simulink subsystem "VehicleBody6DOFSSC"  (R2023b)
settings: Solver=VariableStepAuto  StartTime=0.0  StopTime=10.0  RelTol=1e-3
undefined symbols (not defined in the file): EnvAirDen, PlntVehAeroDragCff, PlntVehAeroFrntArea, PlntVehAeroLiftCff, PlntVehCGHgtAxl, PlntVehDstCGFrntAxl, PlntVehDstCGRearAxl, PlntVehInitLatPos, PlntVehInitVertPos, PlntVehMass, PlntVehMultiBody, PlntVehPitchMomentInertia, PlntVehRollMomentInertia, PlntVehYawMomentInertia, X, Y, Z
libraries: nesl_utility x44, sm_lib x42, sharedtransform x12, fl_lib x4, vehdynlibeomcommon x3, matrix_library x1
(part 2 of 3)

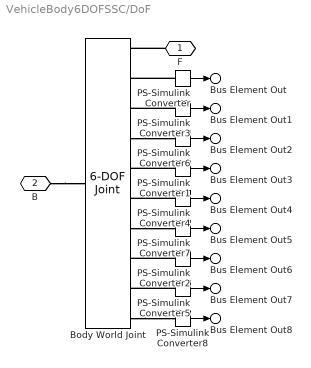
== system VehicleBody6DOFSSC/DoF ==
  Body World Joint : sm_lib/Joints/6-DOF Joint  JointMode=Normal  SenseConstraintForce=off  SenseConstraintForceX=off  SenseConstraintForceY=off  SenseConstraintForceZ=off  SenseConstraintTorque=off  SenseConstraintTorqueX=off  SenseConstraintTorqueY=off  SenseConstraintTorqueZ=off  SenseTotalForce=off  SenseTotalForceX=off  SenseTotalForceY=off  SenseTotalForceZ=off  SenseTotalTorque=off  SenseTotalTorqueX=off  SenseTotalTorqueY=off  SenseTotalTorqueZ=off  CompositeWrenchDir=FollowerOnBase  CompositeWrenchFrame=BaseFrame  PxEquilibriumPosition=0  PxEquilibriumPositionUnits=m  PxSpringStiffness=0  PxSpringStiffnessUnits=N/m  PxDampingCoefficient=0  PxDampingCoefficientUnits=N/(m/s)  PxTorqueActuationMode=NoTorque  PxMotionActuationMode=ComputedMotion  PxSensePosition=on  PxSenseVelocity=on  PxSenseAcceleration=on  PxSenseTorqueForce=off  PxSenseLowerLimitTorqueForce=off  PxSenseUpperLimitTorqueForce=off  PxLowerLimitSpecify=off  PxLowerLimitBound=-1  PxLowerLimitBoundUnits=m  PxLowerLimitStiffness=1e6  PxLowerLimitStiffnessUnits=N/m  PxLowerLimitDamping=1e3  PxLowerLimitDampingUnits=N/(m/s)  PxLowerLimitTransitionRegionWidth=1e-4  PxLowerLimitTransitionRegionWidthUnits=m  PxUpperLimitSpecify=off  PxUpperLimitBound=1  PxUpperLimitBoundUnits=m  PxUpperLimitStiffness=1e6  PxUpperLimitStiffnessUnits=N/m  PxUpperLimitDamping=1e3  PxUpperLimitDampingUnits=N/(m/s)  PxUpperLimitTransitionRegionWidth=1e-4  PxUpperLimitTransitionRegionWidthUnits=m  PxPositionTargetSpecify=on  PxPositionTargetPriority=Low  PxPositionTargetValue=PlntVehInitLongPos  PxPositionTargetValueUnits=m  PxVelocityTargetSpecify=on  PxVelocityTargetPriority=Low  PxVelocityTargetValue=0  PxVelocityTargetValueUnits=m/s  PyEquilibriumPosition=0  PyEquilibriumPositionUnits=m  PySpringStiffness=0  PySpringStiffnessUnits=N/m  PyDampingCoefficient=0  PyDampingCoefficientUnits=N/(m/s)  PyTorqueActuationMode=NoTorque  PyMotionActuationMode=ComputedMotion  PySensePosition=on  PySenseVelocity=on  PySenseAcceleration=on  PySenseTorqueForce=off  PySenseLowerLimitTorqueForce=off  PySenseUpperLimitTorqueForce=off  PyLowerLimitSpecify=off  PyLowerLimitBound=-1  PyLowerLimitBoundUnits=m  PyLowerLimitStiffness=1e6  PyLowerLimitStiffnessUnits=N/m  PyLowerLimitDamping=1e3  PyLowerLimitDampingUnits=N/(m/s)  PyLowerLimitTransitionRegionWidth=1e-4  PyLowerLimitTransitionRegionWidthUnits=m  PyUpperLimitSpecify=off  PyUpperLimitBound=1  PyUpperLimitBoundUnits=m  PyUpperLimitStiffness=1e6  PyUpperLimitStiffnessUnits=N/m  PyUpperLimitDamping=1e3  PyUpperLimitDampingUnits=N/(m/s)  PyUpperLimitTransitionRegionWidth=1e-4  PyUpperLimitTransitionRegionWidthUnits=m  PyPositionTargetSpecify=on  PyPositionTargetPriority=Low  PyPositionTargetValue=-PlntVehInitLatPos  PyPositionTargetValueUnits=m  PyVelocityTargetSpecify=on  PyVelocityTargetPriority=Low  PyVelocityTargetValue=0  PyVelocityTargetValueUnits=m/s  PzEquilibriumPosition=0  PzEquilibriumPositionUnits=m  PzSpringStiffness=0  PzSpringStiffnessUnits=N/m  PzDampingCoefficient=0  PzDampingCoefficientUnits=N/(m/s)  PzTorqueActuationMode=NoTorque  PzMotionActuationMode=ComputedMotion  PzSensePosition=on  PzSenseVelocity=on  PzSenseAcceleration=on  PzSenseTorqueForce=off  PzSenseLowerLimitTorqueForce=off  PzSenseUpperLimitTorqueForce=off  PzLowerLimitSpecify=off  PzLowerLimitBound=-1  PzLowerLimitBoundUnits=m  PzLowerLimitStiffness=1e6  PzLowerLimitStiffnessUnits=N/m  PzLowerLimitDamping=1e3  PzLowerLimitDampingUnits=N/(m/s)  PzLowerLimitTransitionRegionWidth=1e-4  PzLowerLimitTransitionRegionWidthUnits=m  PzUpperLimitSpecify=off  PzUpperLimitBound=1  PzUpperLimitBoundUnits=m  PzUpperLimitStiffness=1e6  PzUpperLimitStiffnessUnits=N/m  PzUpperLimitDamping=1e3  PzUpperLimitDampingUnits=N/(m/s)  PzUpperLimitTransitionRegionWidth=1e-4  PzUpperLimitTransitionRegionWidthUnits=m  PzPositionTargetSpecify=on  PzPositionTargetPriority=Low  PzPositionTargetValue=-PlntVehInitVertPos*0  PzPositionTargetValueUnits=m  PzVelocityTargetSpecify=on  PzVelocityTargetPriority=Low  PzVelocityTargetValue=0  PzVelocityTargetValueUnits=m/s  SphEqPosRotationMethod=None  SphEqPosRotationAngleUnits=deg  SphEqPosRotationStandardAxis=+Z  SphEqPosRotationAngle=0.0  SphEqPosRotationArbitraryAxis=[0 0 1]  SphEqPosFollAlignAxisA=+X  SphEqPosBaseAlignAxisA=+Y  SphEqPosFollAlignAxisB=+Y  SphEqPosBaseAlignAxisB=+Z  SphEqPosRotationSequenceAxes=FollowerAxes  SphEqPosRotationSequence=XYX  SphEqPosRotationSequenceAngles=[0 0 0]  SphEqPosRotationSequenceAnglesUnits=deg  SphEqPosRotationMatrix=[1 0 0; 0 1 0; 0 0 1]  SphEqPosQuaternion=[1 0 0 0]  SphSpringStiffness=0  SphSpringStiffnessUnits=N*m/deg  SphDampingCoefficient=0  SphDampingCoefficientUnits=N*m/(deg/s)  SphActuateTorqueX=off  SphActuateTorqueY=off  SphActuateTorqueZ=off  SphActuateTorque=off  SphTorqueActuationMode=NoTorque  SphMotionActuationMode=ComputedMotion  SphActuationFrame=BaseFrame  SphSensePosition=off  SphSenseVelocityX=off  SphSenseVelocityY=off  SphSenseVelocityZ=off  SphSenseVelocity=off  SphSenseAccelerationX=off  SphSenseAccelerationY=off  SphSenseAccelerationZ=off  SphSenseAcceleration=off  SphSenseTorqueX=off  SphSenseTorqueY=off  SphSenseTorqueZ=off  SphSenseTorqueForce=off  SphSenseLowerLimitTorqueMag=off  SphSenseUpperLimitTorqueMag=off  SphSensingFrame=BaseFrame  SphLowerLimitSpecify=off  SphLowerLimitBound=15  SphLowerLimitBoundUnits=deg  SphLowerLimitStiffness=1e4  SphLowerLimitStiffnessUnits=N*m/deg  SphLowerLimitDamping=10  SphLowerLimitDampingUnits=N*m/(deg/s)  SphLowerLimitTransitionRegionWidth=0.1  SphLowerLimitTransitionRegionWidthUnits=deg  SphUpperLimitSpecify=off  SphUpperLimitBound=45  SphUpperLimitBoundUnits=deg  SphUpperLimitStiffness=1e4  SphUpperLimitStiffnessUnits=N*m/deg  SphUpperLimitDamping=10  SphUpperLimitDampingUnits=N*m/(deg/s)  SphUpperLimitTransitionRegionWidth=0.1  SphUpperLimitTransitionRegionWidthUnits=deg  SphPositionTargetRotationMethod=RotationSequence  SphPositionTargetRotationAngleUnits=deg  SphPositionTargetRotationStandardAxis=+Z  SphPositionTargetRotationAngle=0.0  SphPositionTargetRotationArbitraryAxis=[0 0 1]  SphPositionTargetFollAlignAxisA=+X  SphPositionTargetBaseAlignAxisA=+Y  SphPositionTargetFollAlignAxisB=+Y  SphPositionTargetBaseAlignAxisB=+Z  SphPositionTargetRotationSequenceAxes=BaseAxes  SphPositionTargetRotationSequence=XYZ  SphPositionTargetRotationSequenceAngles=[0 0 0]  SphPositionTargetRotationSequenceAnglesUnits=deg  SphPositionTargetRotationMatrix=[1 0 0; 0 1 0; 0 0 1]  SphPositionTargetQuaternion=[1 0 0 0]  SphPositionTargetSpecify=on  SphPositionTargetPriority=Low  SphVelocityTargetValue=[0 0 0]  SphVelocityTargetValueUnits=deg/s  SphVelocityTargetSpecify=off  SphVelocityTargetPriority=High  SphVelocityTargetInFollowerFrame=on
  PS-Simulink Converter : nesl_utility/PS-Simulink Converter  PhysicalDomain=network_engine_domain  SubClassName=ps_output  LeftPortType=input  RightPortType=output  PseudoPeriodic=off  Frequencies=[]  VectorFormat=1-D array  Unit=m  AffineConversion=off
  PS-Simulink Converter1 : nesl_utility/PS-Simulink Converter  PhysicalDomain=network_engine_domain  SubClassName=ps_output  LeftPortType=input  RightPortType=output  PseudoPeriodic=off  Frequencies=[]  VectorFormat=1-D array  Unit=m  AffineConversion=off
  PS-Simulink Converter2 : nesl_utility/PS-Simulink Converter  PhysicalDomain=network_engine_domain  SubClassName=ps_output  LeftPortType=input  RightPortType=output  PseudoPeriodic=off  Frequencies=[]  VectorFormat=1-D array  Unit=m  AffineConversion=off
  PS-Simulink Converter3 : nesl_utility/PS-Simulink Converter  PhysicalDomain=network_engine_domain  SubClassName=ps_output  LeftPortType=input  RightPortType=output  PseudoPeriodic=off  Frequencies=[]  VectorFormat=1-D array  Unit=m/s  AffineConversion=off
  PS-Simulink Converter4 : nesl_utility/PS-Simulink Converter  PhysicalDomain=network_engine_domain  SubClassName=ps_output  LeftPortType=input  RightPortType=output  PseudoPeriodic=off  Frequencies=[]  VectorFormat=1-D array  Unit=m/s  AffineConversion=off
  PS-Simulink Converter5 : nesl_utility/PS-Simulink Converter  PhysicalDomain=network_engine_domain  SubClassName=ps_output  LeftPortType=input  RightPortType=output  PseudoPeriodic=off  Frequencies=[]  VectorFormat=1-D array  Unit=m/s  AffineConversion=off
  PS-Simulink Converter6 : nesl_utility/PS-Simulink Converter  PhysicalDomain=network_engine_domain  SubClassName=ps_output  LeftPortType=input  RightPortType=output  PseudoPeriodic=off  Frequencies=[]  VectorFormat=1-D array  Unit=m/s^2  AffineConversion=off
  PS-Simulink Converter7 : nesl_utility/PS-Simulink Converter  PhysicalDomain=network_engine_domain  SubClassName=ps_output  LeftPortType=input  RightPortType=output  PseudoPeriodic=off  Frequencies=[]  VectorFormat=1-D array  Unit=m/s^2  AffineConversion=off
  PS-Simulink Converter8 : nesl_utility/PS-Simulink Converter  PhysicalDomain=network_engine_domain  SubClassName=ps_output  LeftPortType=input  RightPortType=output  PseudoPeriodic=off  Frequencies=[]  VectorFormat=1-D array  Unit=m/s^2  AffineConversion=off
  F : PMIOPort  Side=Left
  B : PMIOPort  Port=2  Side=Right
  Bus Element Out : Outport  VectorParamsAs1DForOutWhenUnconnected=off  PortName=World  Element=x
  Bus Element Out3 : Outport  VectorParamsAs1DForOutWhenUnconnected=off  PortName=World  Element=y
  Bus Element Out6 : Outport  VectorParamsAs1DForOutWhenUnconnected=off  PortName=World  Element=z
  Bus Element Out1 : Outport  VectorParamsAs1DForOutWhenUnconnected=off  PortName=World  Element=vx
  Bus Element Out4 : Outport  VectorParamsAs1DForOutWhenUnconnected=off  PortName=World  Element=vy
  Bus Element Out7 : Outport  VectorParamsAs1DForOutWhenUnconnected=off  PortName=World  Element=vz
  Bus Element Out2 : Outport  VectorParamsAs1DForOutWhenUnconnected=off  PortName=World  Element=gx
  Bus Element Out5 : Outport  VectorParamsAs1DForOutWhenUnconnected=off  PortName=World  Element=gy
  Bus Element Out8 : Outport  VectorParamsAs1DForOutWhenUnconnected=off  PortName=World  Element=gz
  wires:
  PS-Simulink Converter8/1 -> Bus Element Out8/1
  PS-Simulink Converter7/1 -> Bus Element Out5/1
  PS-Simulink Converter5/1 -> Bus Element Out7/1
  PS-Simulink Converter4/1 -> Bus Element Out4/1
  PS-Simulink Converter3/1 -> Bus Element Out1/1
  PS-Simulink Converter6/1 -> Bus Element Out2/1
  PS-Simulink Converter2/1 -> Bus Element Out6/1
  PS-Simulink Converter/1 -> Bus Element Out/1
  PS-Simulink Converter1/1 -> Bus Element Out3/1
  connections:
  PS-Simulink Converter5/LConn1 -- Body World Joint/RConn9
  Body World Joint/RConn7 -- PS-Simulink Converter7/LConn1
  PS-Simulink Converter1/LConn1 -- Body World Joint/RConn5
  PS-Simulink Converter4/LConn1 -- Body World Joint/RConn6
  PS-Simulink Converter3/LConn1 -- Body World Joint/RConn3
  PS-Simulink Converter/LConn1 -- Body World Joint/RConn2
  B/RConn1 -- Body World Joint/LConn1
  Body World Joint/RConn4 -- PS-Simulink Converter6/LConn1
  Body World Joint/RConn10 -- PS-Simulink Converter8/LConn1
  F/RConn1 -- Body World Joint/RConn1
  PS-Simulink Converter2/LConn1 -- Body World Joint/RConn8

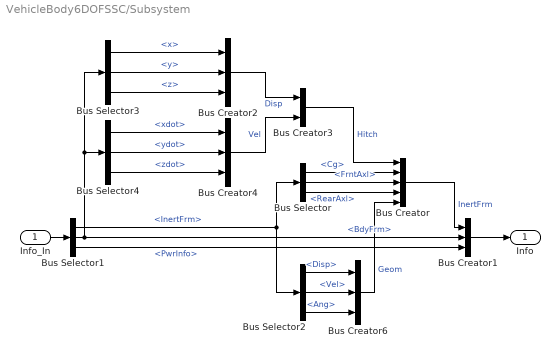
== system VehicleBody6DOFSSC/Subsystem ==
  Info_In : Inport
  Bus Creator : BusCreator  Inputs=5
  Bus Creator{1..2,4,6} (4 alike) : BusCreator  Inputs=3
  Bus Creator3 : BusCreator  Inputs=2
  Bus Selector : BusSelector  OutputSignals=Cg,FrntAxl,RearAxl
  Bus Selector1 : BusSelector  OutputSignals=InertFrm,BdyFrm,PwrInfo
  Bus Selector2 : BusSelector  OutputSignals=Cg.Disp,Cg.Vel,Cg.Ang
  Bus Selector3 : BusSelector  OutputSignals=Cg.Disp.x,Cg.Disp.y,Cg.Disp.z
  Bus Selector4 : BusSelector  OutputSignals=Cg.Vel.xdot,Cg.Vel.ydot,Cg.Vel.zdot
  Info : Outport
  wires:
  Bus Selector4/3 -> Bus Creator4/3  "<zdot>"
  Bus Selector4/2 -> Bus Creator4/2  "<ydot>"
  Bus Selector4/1 -> Bus Creator4/1  "<xdot>"
  Bus Selector3/3 -> Bus Creator2/3  "<z>"
  Bus Selector3/2 -> Bus Creator2/2  "<y>"
  Bus Selector3/1 -> Bus Creator2/1  "<x>"
  Bus Selector2/3 -> Bus Creator6/3  "<Ang>"
  Bus Selector2/2 -> Bus Creator6/2  "<Vel>"
  Bus Selector2/1 -> Bus Creator6/1  "<Disp>"
  Bus Creator6/1 -> Bus Creator/5  "Geom"
  Bus Selector1/2 -> Bus Creator1/2, Bus Selector4/1, Bus Selector3/1  "<BdyFrm>"
  Info_In/1 -> Bus Selector1/1
  Bus Creator/1 -> Bus Creator1/1  "InertFrm"
  Bus Selector/3 -> Bus Creator/4  "<RearAxl>"
  Bus Selector1/1 -> Bus Selector/1, Bus Selector2/1  "<InertFrm>"
  Bus Creator1/1 -> Info/1
  Bus Creator3/1 -> Bus Creator/1  "Hitch"
  Bus Selector1/3 -> Bus Creator1/3  "<PwrInfo>"
  Bus Selector/1 -> Bus Creator/2  "<Cg>"
  Bus Selector/2 -> Bus Creator/3  "<FrntAxl>"
  Bus Creator4/1 -> Bus Creator3/2  "Vel"
  Bus Creator2/1 -> Bus Creator3/1  "Disp"

== system VehicleBody6DOFSSC/World ==
  MechanismConfiguration : sm_lib/Utilities/Mechanism Configuration  UniformGravity=Constant  GravityVector=[0 0 -9.80665]  GravityVectorUnits=m/s^2  LinearizationDelta=0.001  JointModeTransitionNonlinearIterations=2
  World Frame : sm_lib/Frames and Transforms/World Frame
  W : PMIOPort  Side=Right
  connections:
  MechanismConfiguration/RConn1 -- W/RConn1 -- World Frame/RConn1

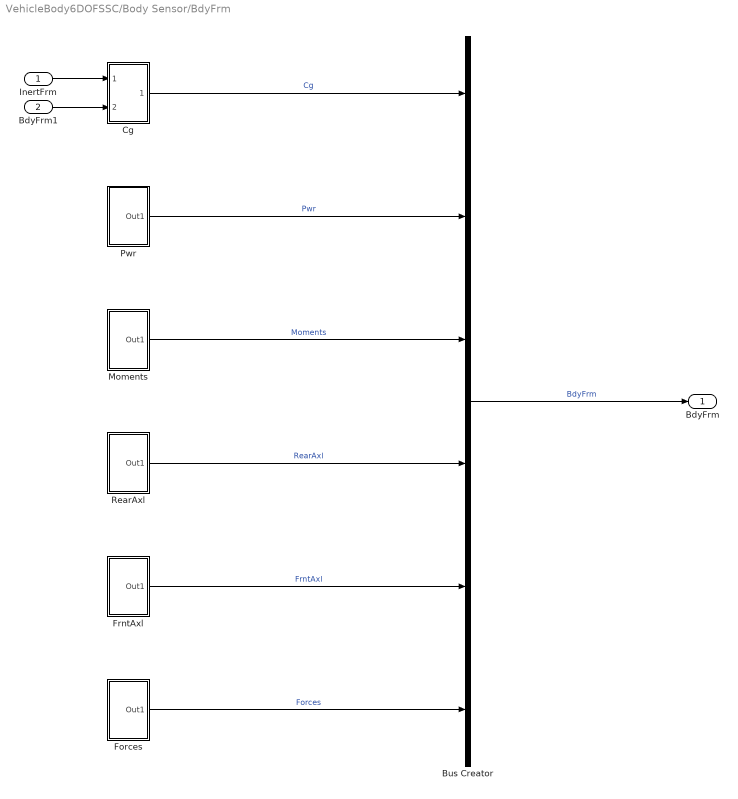
== system VehicleBody6DOFSSC/Body Sensor/BdyFrm ==
  InertFrm : Inport
  BdyFrm1 : Inport  Port=2
  Bus Creator : BusCreator  Inputs=6
  Cg : Subsystem
  Forces : Subsystem
  FrntAxl : Subsystem
  Moments : Subsystem
  Pwr : Subsystem
  RearAxl : Subsystem
  BdyFrm : Outport
  wires:
  Bus Creator/1 -> BdyFrm/1  "BdyFrm"
  Pwr/1(Out1) -> Bus Creator/2  "Pwr"
  Moments/1(Out1) -> Bus Creator/3  "Moments"
  RearAxl/1(Out1) -> Bus Creator/4  "RearAxl"
  FrntAxl/1(Out1) -> Bus Creator/5  "FrntAxl"
  Forces/1(Out1) -> Bus Creator/6  "Forces"
  Cg/1(Out1) -> Bus Creator/1  "Cg"
  BdyFrm1/1 -> Cg/2(BdyFrm)
  InertFrm/1 -> Cg/1(InertFrm)

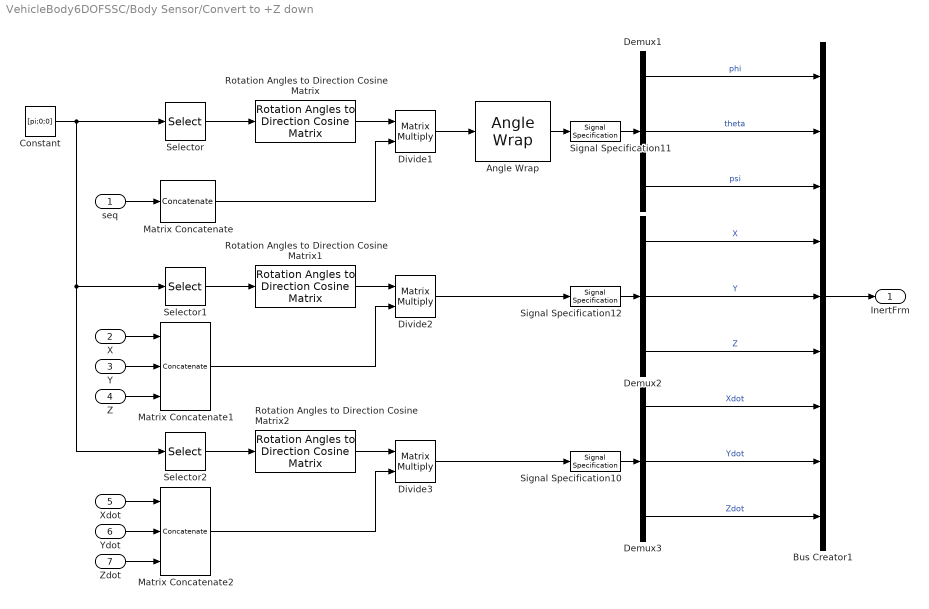
== system VehicleBody6DOFSSC/Body Sensor/Convert to +Z down ==
  seq : Inport
  X : Inport  Port=2
  Y : Inport  Port=3
  Z : Inport  Port=4
  Xdot : Inport  Port=5
  Ydot : Inport  Port=6
  Zdot : Inport  Port=7
  Angle Wrap : vehdynlibeomcommon/6 DOF Generic Vehicle Body/SignalCollection/Angle Wrap  SystemSampleTime=-1  VariantControl=Variant1  LabelModeActiveChoice=Unwrap  VariantActivationTime=update diagram  AllowFlexibleInterface=on  Latency=0  AutoFrameSizeCalculation=off
      link override Unwrap/Unwrap: aMode=6
  Bus Creator1 : BusCreator  Inputs=9
  Constant : Constant  Value=[pi;0;0]
  Demux1 : Demux  Outputs=3
  Demux2 : Demux  Outputs=3
  Demux3 : Demux  Outputs=3
  Divide1 : Product  Inputs=**  Multiplication=Matrix(*)
  Divide2 : Product  Inputs=**  Multiplication=Matrix(*)
  Divide3 : Product  Inputs=**  Multiplication=Matrix(*)
  Matrix Concatenate : Concatenate  NumInputs=1  Mode=Multidimensional array
  Matrix Concatenate1 : Concatenate  NumInputs=3  Mode=Multidimensional array
  Matrix Concatenate2 : Concatenate  NumInputs=3  Mode=Multidimensional array
  Rotation Angles to Direction Cosine Matrix : sharedtransform/Rotation Angles to Direction Cosine Matrix  rotationOrder=ZYX  aMode=2
  Rotation Angles to Direction Cosine Matrix1 : sharedtransform/Rotation Angles to Direction Cosine Matrix  rotationOrder=ZYX  aMode=2
  Rotation Angles to Direction Cosine Matrix2 : sharedtransform/Rotation Angles to Direction Cosine Matrix  rotationOrder=ZYX  aMode=2
  Selector : Selector  InputPortWidth=3  IndexOptions=Index vector (dialog)  Indices=[3 2 1]  OutputSizes=1
  Selector1 : Selector  InputPortWidth=3  IndexOptions=Index vector (dialog)  Indices=[3 2 1]  OutputSizes=1
  Selector2 : Selector  InputPortWidth=3  IndexOptions=Index vector (dialog)  Indices=[3 2 1]  OutputSizes=1
  Signal Specification10 : SignalSpecification  Unit=m/s
  Signal Specification11 : SignalSpecification  Unit=rad
  Signal Specification12 : SignalSpecification  Unit=m
  InertFrm : Outport
  wires:
  Selector/1 -> Rotation Angles to Direction Cosine Matrix/1
  Rotation Angles to Direction Cosine Matrix/1 -> Divide1/1
  Divide1/1 -> Angle Wrap/1
  Demux2/2 -> Bus Creator1/5  "Y"
  Demux3/3 -> Bus Creator1/9  "Zdot"
  Demux1/2 -> Bus Creator1/2  "theta"
  Demux2/3 -> Bus Creator1/6  "Z"
  Demux3/2 -> Bus Creator1/8  "Ydot"
  Demux3/1 -> Bus Creator1/7  "Xdot"
  Demux2/1 -> Bus Creator1/4  "X"
  Demux1/1 -> Bus Creator1/1  "phi"
  Demux1/3 -> Bus Creator1/3  "psi"
  seq/1 -> Matrix Concatenate/1
  Matrix Concatenate/1 -> Divide1/2
  Matrix Concatenate1/1 -> Divide2/2
  X/1 -> Matrix Concatenate1/1
  Rotation Angles to Direction Cosine Matrix1/1 -> Divide2/1
  Selector1/1 -> Rotation Angles to Direction Cosine Matrix1/1
  Divide2/1 -> Signal Specification12/1
  Y/1 -> Matrix Concatenate1/2
  Z/1 -> Matrix Concatenate1/3
  Zdot/1 -> Matrix Concatenate2/3
  Ydot/1 -> Matrix Concatenate2/2
  Selector2/1 -> Rotation Angles to Direction Cosine Matrix2/1
  Rotation Angles to Direction Cosine Matrix2/1 -> Divide3/1
  Constant/1 -> Selector2/1, Selector1/1, Selector/1
  Xdot/1 -> Matrix Concatenate2/1
  Matrix Concatenate2/1 -> Divide3/2
  Divide3/1 -> Signal Specification10/1
  Bus Creator1/1 -> InertFrm/1
  Angle Wrap/1 -> Signal Specification11/1
  Signal Specification10/1 -> Demux3/1
  Signal Specification11/1 -> Demux1/1
  Signal Specification12/1 -> Demux2/1

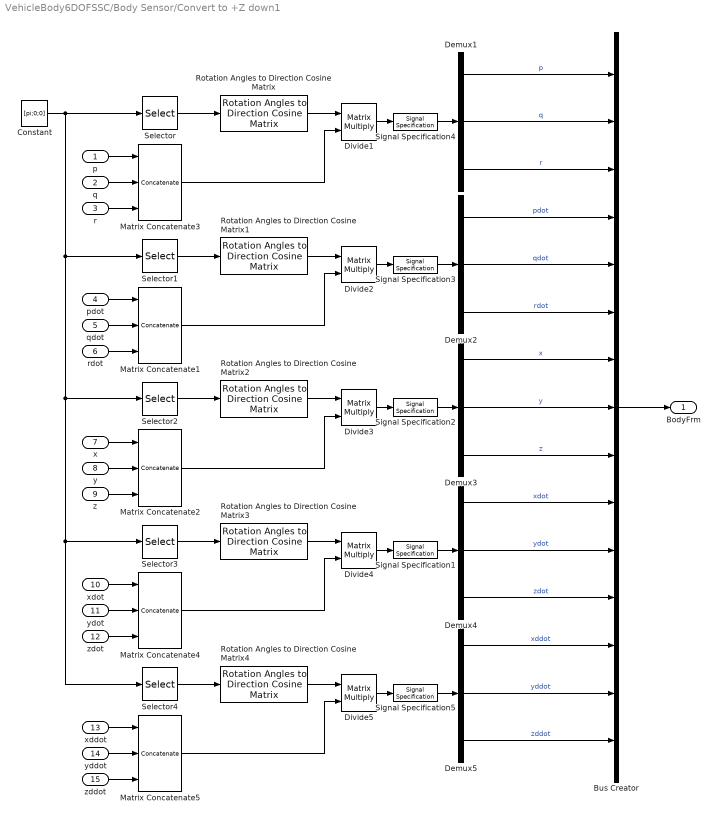
== system VehicleBody6DOFSSC/Body Sensor/Convert to +Z down1 ==
  p : Inport
  q : Inport  Port=2
  r : Inport  Port=3
  pdot : Inport  Port=4
  qdot : Inport  Port=5
  rdot : Inport  Port=6
  x : Inport  Port=7
  y : Inport  Port=8
  z : Inport  Port=9
  xdot : Inport  Port=10
  ydot : Inport  Port=11
  zdot : Inport  Port=12
  xddot : Inport  Port=13
  yddot : Inport  Port=14
  zddot : Inport  Port=15
  Bus Creator : BusCreator  Inputs=15
  Constant : Constant  Value=[pi;0;0]
  Demux{1..5} (5 alike) : Demux  Outputs=3
  Divide{1..5} (5 alike) : Product  Inputs=**  Multiplication=Matrix(*)
  Matrix Concatenate{1..5} (5 alike) : Concatenate  NumInputs=3  Mode=Multidimensional array
  Rotation Angles to Direction Cosine Matrix{,1..4} (5 alike) : sharedtransform/Rotation Angles to Direction Cosine Matrix  rotationOrder=ZYX  aMode=2
  Selector{,1..4} (5 alike) : Selector  InputPortWidth=3  IndexOptions=Index vector (dialog)  Indices=[3 2 1]  OutputSizes=1
  Signal Specification1 : SignalSpecification  Unit=m/s
  Signal Specification2 : SignalSpecification  Unit=m
  Signal Specification3 : SignalSpecification  Unit=rad/s^2
  Signal Specification4 : SignalSpecification  Unit=rad/s
  Signal Specification5 : SignalSpecification  Unit=m/s^2
  BodyFrm : Outport
  wires:
  Divide3/1 -> Signal Specification2/1
  Matrix Concatenate2/1 -> Divide3/2
  x/1 -> Matrix Concatenate2/1
  Rotation Angles to Direction Cosine Matrix2/1 -> Divide3/1
  Selector2/1 -> Rotation Angles to Direction Cosine Matrix2/1
  y/1 -> Matrix Concatenate2/2
  z/1 -> Matrix Concatenate2/3
  rdot/1 -> Matrix Concatenate1/3
  qdot/1 -> Matrix Concatenate1/2
  Divide2/1 -> Signal Specification3/1
  Selector1/1 -> Rotation Angles to Direction Cosine Matrix1/1
  Rotation Angles to Direction Cosine Matrix1/1 -> Divide2/1
  pdot/1 -> Matrix Concatenate1/1
  Matrix Concatenate1/1 -> Divide2/2
  Divide1/1 -> Signal Specification4/1
  Rotation Angles to Direction Cosine Matrix/1 -> Divide1/1
  Selector/1 -> Rotation Angles to Direction Cosine Matrix/1
  Bus Creator/1 -> BodyFrm/1
  Demux1/1 -> Bus Creator/1  "p"
  Demux1/2 -> Bus Creator/2  "q"
  Demux1/3 -> Bus Creator/3  "r"
  Demux2/1 -> Bus Creator/4  "pdot"
  Demux2/2 -> Bus Creator/5  "qdot"
  Demux2/3 -> Bus Creator/6  "rdot"
  Demux3/1 -> Bus Creator/7  "x"
  Demux3/2 -> Bus Creator/8  "y"
  Demux3/3 -> Bus Creator/9  "z"
  Demux4/1 -> Bus Creator/10  "xdot"
  Demux4/2 -> Bus Creator/11  "ydot"
  Demux4/3 -> Bus Creator/12  "zdot"
  Demux5/1 -> Bus Creator/13  "xddot"
  Demux5/2 -> Bus Creator/14  "yddot"
  Demux5/3 -> Bus Creator/15  "zddot"
  Matrix Concatenate3/1 -> Divide1/2
  p/1 -> Matrix Concatenate3/1
  r/1 -> Matrix Concatenate3/3
  q/1 -> Matrix Concatenate3/2
  zdot/1 -> Matrix Concatenate4/3
  ydot/1 -> Matrix Concatenate4/2
  Selector3/1 -> Rotation Angles to Direction Cosine Matrix3/1
  Rotation Angles to Direction Cosine Matrix3/1 -> Divide4/1
  xdot/1 -> Matrix Concatenate4/1
  Matrix Concatenate4/1 -> Divide4/2
  Divide4/1 -> Signal Specification1/1
  Matrix Concatenate5/1 -> Divide5/2
  xddot/1 -> Matrix Concatenate5/1
  Constant/1 -> Selector/1, Selector1/1, Selector4/1, Selector3/1, Selector2/1
  Rotation Angles to Direction Cosine Matrix4/1 -> Divide5/1
  Selector4/1 -> Rotation Angles to Direction Cosine Matrix4/1
  yddot/1 -> Matrix Concatenate5/2
  zddot/1 -> Matrix Concatenate5/3
  Divide5/1 -> Signal Specification5/1
  Signal Specification5/1 -> Demux5/1
  Signal Specification1/1 -> Demux4/1
  Signal Specification2/1 -> Demux3/1
  Signal Specification3/1 -> Demux2/1
  Signal Specification4/1 -> Demux1/1

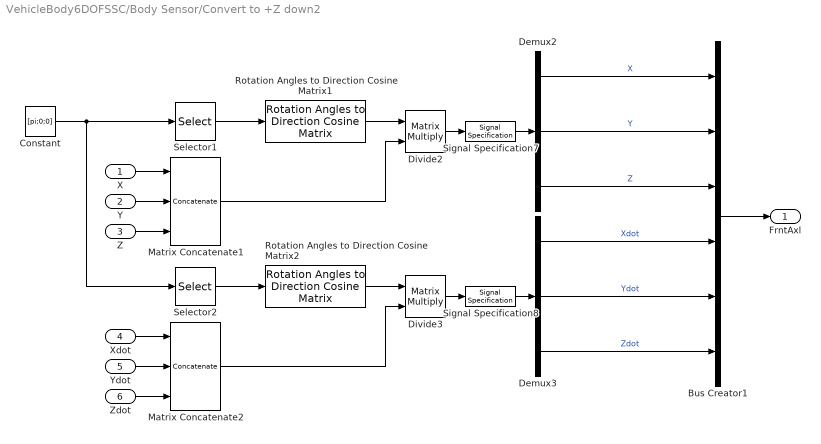
== system VehicleBody6DOFSSC/Body Sensor/Convert to +Z down2 ==
  X : Inport
  Y : Inport  Port=2
  Z : Inport  Port=3
  Xdot : Inport  Port=4
  Ydot : Inport  Port=5
  Zdot : Inport  Port=6
  Bus Creator1 : BusCreator  Inputs=6
  Constant : Constant  Value=[pi;0;0]
  Demux2 : Demux  Outputs=3
  Demux3 : Demux  Outputs=3
  Divide2 : Product  Inputs=**  Multiplication=Matrix(*)
  Divide3 : Product  Inputs=**  Multiplication=Matrix(*)
  Matrix Concatenate1 : Concatenate  NumInputs=3  Mode=Multidimensional array
  Matrix Concatenate2 : Concatenate  NumInputs=3  Mode=Multidimensional array
  Rotation Angles to Direction Cosine Matrix1 : sharedtransform/Rotation Angles to Direction Cosine Matrix  rotationOrder=ZYX  aMode=2
  Rotation Angles to Direction Cosine Matrix2 : sharedtransform/Rotation Angles to Direction Cosine Matrix  rotationOrder=ZYX  aMode=2
  Selector1 : Selector  InputPortWidth=3  IndexOptions=Index vector (dialog)  Indices=[3 2 1]  OutputSizes=1
  Selector2 : Selector  InputPortWidth=3  IndexOptions=Index vector (dialog)  Indices=[3 2 1]  OutputSizes=1
  Signal Specification7 : SignalSpecification  Unit=m
  Signal Specification8 : SignalSpecification  Unit=m/s
  FrntAxl : Outport
  wires:
  Bus Creator1/1 -> FrntAxl/1
  Divide3/1 -> Signal Specification8/1
  Matrix Concatenate2/1 -> Divide3/2
  Xdot/1 -> Matrix Concatenate2/1
  Constant/1 -> Selector1/1, Selector2/1
  Rotation Angles to Direction Cosine Matrix2/1 -> Divide3/1
  Selector2/1 -> Rotation Angles to Direction Cosine Matrix2/1
  Ydot/1 -> Matrix Concatenate2/2
  Zdot/1 -> Matrix Concatenate2/3
  Z/1 -> Matrix Concatenate1/3
  Y/1 -> Matrix Concatenate1/2
  Divide2/1 -> Signal Specification7/1
  Selector1/1 -> Rotation Angles to Direction Cosine Matrix1/1
  Rotation Angles to Direction Cosine Matrix1/1 -> Divide2/1
  X/1 -> Matrix Concatenate1/1
  Matrix Concatenate1/1 -> Divide2/2
  Demux2/1 -> Bus Creator1/1  "X"
  Demux3/1 -> Bus Creator1/4  "Xdot"
  Demux3/2 -> Bus Creator1/5  "Ydot"
  Demux2/3 -> Bus Creator1/3  "Z"
  Demux3/3 -> Bus Creator1/6  "Zdot"
  Demux2/2 -> Bus Creator1/2  "Y"
  Signal Specification7/1 -> Demux2/1
  Signal Specification8/1 -> Demux3/1

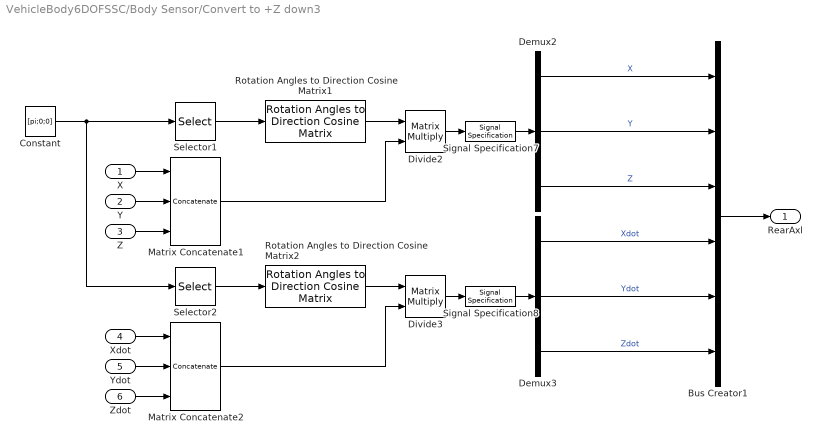
== system VehicleBody6DOFSSC/Body Sensor/Convert to +Z down3 ==
  X : Inport
  Y : Inport  Port=2
  Z : Inport  Port=3
  Xdot : Inport  Port=4
  Ydot : Inport  Port=5
  Zdot : Inport  Port=6
  Bus Creator1 : BusCreator  Inputs=6
  Constant : Constant  Value=[pi;0;0]
  Demux2 : Demux  Outputs=3
  Demux3 : Demux  Outputs=3
  Divide2 : Product  Inputs=**  Multiplication=Matrix(*)
  Divide3 : Product  Inputs=**  Multiplication=Matrix(*)
  Matrix Concatenate1 : Concatenate  NumInputs=3  Mode=Multidimensional array
  Matrix Concatenate2 : Concatenate  NumInputs=3  Mode=Multidimensional array
  Rotation Angles to Direction Cosine Matrix1 : sharedtransform/Rotation Angles to Direction Cosine Matrix  rotationOrder=ZYX  aMode=2
  Rotation Angles to Direction Cosine Matrix2 : sharedtransform/Rotation Angles to Direction Cosine Matrix  rotationOrder=ZYX  aMode=2
  Selector1 : Selector  InputPortWidth=3  IndexOptions=Index vector (dialog)  Indices=[3 2 1]  OutputSizes=1
  Selector2 : Selector  InputPortWidth=3  IndexOptions=Index vector (dialog)  Indices=[3 2 1]  OutputSizes=1
  Signal Specification7 : SignalSpecification  Unit=m
  Signal Specification8 : SignalSpecification  Unit=m/s
  RearAxl : Outport
  wires:
  Demux2/2 -> Bus Creator1/2  "Y"
  Demux3/3 -> Bus Creator1/6  "Zdot"
  Demux2/3 -> Bus Creator1/3  "Z"
  Demux3/2 -> Bus Creator1/5  "Ydot"
  Demux3/1 -> Bus Creator1/4  "Xdot"
  Demux2/1 -> Bus Creator1/1  "X"
  Matrix Concatenate1/1 -> Divide2/2
  X/1 -> Matrix Concatenate1/1
  Rotation Angles to Direction Cosine Matrix1/1 -> Divide2/1
  Selector1/1 -> Rotation Angles to Direction Cosine Matrix1/1
  Divide2/1 -> Signal Specification7/1
  Y/1 -> Matrix Concatenate1/2
  Z/1 -> Matrix Concatenate1/3
  Zdot/1 -> Matrix Concatenate2/3
  Ydot/1 -> Matrix Concatenate2/2
  Selector2/1 -> Rotation Angles to Direction Cosine Matrix2/1
  Rotation Angles to Direction Cosine Matrix2/1 -> Divide3/1
  Constant/1 -> Selector2/1, Selector1/1
  Xdot/1 -> Matrix Concatenate2/1
  Matrix Concatenate2/1 -> Divide3/2
  Divide3/1 -> Signal Specification8/1
  Bus Creator1/1 -> RearAxl/1
  Signal Specification7/1 -> Demux2/1
  Signal Specification8/1 -> Demux3/1

== system VehicleBody6DOFSSC/Body Sensor/InertFrm ==
  FrntAxl1 : Inport
  RearAxl1 : Inport  Port=2
  CG : Inport  Port=3
  Bus Creator : BusCreator  Inputs=5
  Cg : Subsystem
  FrntAxl : Subsystem
  Geom : Subsystem
  Hitch : Subsystem
  RearAxl : Subsystem
  InertFrm : Outport
  wires:
  CG/1 -> Geom/1(In), Cg/1(In)
  Bus Creator/1 -> InertFrm/1  "InertFrm"
  Cg/1(Out1) -> Bus Creator/5  "Cg"
  Geom/1(Out1) -> Bus Creator/1  "Geom"
  FrntAxl/1(Out1) -> Bus Creator/2  "FrntAxl"
  RearAxl/1(Out1) -> Bus Creator/3  "RearAxl"
  Hitch/1(Out1) -> Bus Creator/4  "Hitch"
  FrntAxl1/1 -> FrntAxl/1(In)
  RearAxl1/1 -> RearAxl/1(RearAxl1)

== system VehicleBody6DOFSSC/Body Sensor/PwrInfo ==
  Bus Creator : BusCreator  Inputs=3
  vehBus_Values_PwrInfo_PwrNotTrnsfrd : Subsystem
  vehBus_Values_PwrInfo_PwrStored : Subsystem
  vehBus_Values_PwrInfo_PwrTrnsfrd : Subsystem
  PwrInfo : Outport
  wires:
  vehBus_Values_PwrInfo_PwrTrnsfrd/1(Out1) -> Bus Creator/1  "PwrTrnsfrd"
  vehBus_Values_PwrInfo_PwrStored/1(Out1) -> Bus Creator/2  "PwrStored"
  vehBus_Values_PwrInfo_PwrNotTrnsfrd/1(Out1) -> Bus Creator/3  "PwrNotTrnsfrd"
  Bus Creator/1 -> PwrInfo/1  "PwrInfo"

== system VehicleBody6DOFSSC/Body Sensor/BdyFrm/Cg ==
  InertFrm : Inport
  BdyFrm : Inport  Port=2
  Bus Creator : BusCreator  Inputs=5
  vehBus_Values_BdyFrm_Cg_Acc : Subsystem
  vehBus_Values_BdyFrm_Cg_AngAcc : Subsystem
  vehBus_Values_BdyFrm_Cg_AngVel : Subsystem
  vehBus_Values_BdyFrm_Cg_Disp : Subsystem
  vehBus_Values_BdyFrm_Cg_Vel : Subsystem
  Out1 : Outport
  wires:
  vehBus_Values_BdyFrm_Cg_Vel/1(Out1) -> Bus Creator/4  "Vel"
  vehBus_Values_BdyFrm_Cg_AngVel/1(Out2) -> Bus Creator/1  "AngVel"
  vehBus_Values_BdyFrm_Cg_Acc/1(Out2) -> Bus Creator/3  "Acc"
  Bus Creator/1 -> Out1/1
  BdyFrm/1 -> vehBus_Values_BdyFrm_Cg_Vel/1(In), vehBus_Values_BdyFrm_Cg_Disp/1(In), vehBus_Values_BdyFrm_Cg_Acc/1(BdyFrm), vehBus_Values_BdyFrm_Cg_AngAcc/1(In), vehBus_Values_BdyFrm_Cg_AngVel/1(In)
  InertFrm/1 -> vehBus_Values_BdyFrm_Cg_Acc/2(InertFrm)
  vehBus_Values_BdyFrm_Cg_Disp/1(Out2) -> Bus Creator/5  "Disp"
  vehBus_Values_BdyFrm_Cg_AngAcc/1(Out2) -> Bus Creator/2  "AngAcc"

== system VehicleBody6DOFSSC/Body Sensor/BdyFrm/Forces ==
  Bus Creator : BusCreator  Inputs=8
  vehBus_Values_BdyFrm_Forces_Body : Subsystem
  vehBus_Values_BdyFrm_Forces_Drag : Subsystem
  vehBus_Values_BdyFrm_Forces_Ext : Subsystem
  vehBus_Values_BdyFrm_Forces_FrntAxl : Subsystem
  vehBus_Values_BdyFrm_Forces_Grvty : Subsystem
  vehBus_Values_BdyFrm_Forces_RearAxl : Subsystem
  vehBus_Values_BdyFrm_Forces_Tires_FrntTire : Subsystem
  vehBus_Values_BdyFrm_Forces_Tires_RearTire : Subsystem
  Out1 : Outport
  wires:
  vehBus_Values_BdyFrm_Forces_FrntAxl/1(Out1) -> Bus Creator/1  "FrntAxl"
  vehBus_Values_BdyFrm_Forces_Drag/1(Out1) -> Bus Creator/2  "Drag"
  vehBus_Values_BdyFrm_Forces_Grvty/1(Out1) -> Bus Creator/8  "Grvty"
  vehBus_Values_BdyFrm_Forces_Tires_RearTire/1(Out1) -> Bus Creator/5  "RearTire"
  vehBus_Values_BdyFrm_Forces_Body/1(Out1) -> Bus Creator/6  "Body"
  vehBus_Values_BdyFrm_Forces_Tires_FrntTire/1(Out1) -> Bus Creator/4  "FrntTire"
  vehBus_Values_BdyFrm_Forces_RearAxl/1(Out1) -> Bus Creator/3  "RearAxl"
  vehBus_Values_BdyFrm_Forces_Ext/1(Out1) -> Bus Creator/7  "Ext"
  Bus Creator/1 -> Out1/1

== system VehicleBody6DOFSSC/Body Sensor/BdyFrm/FrntAxl ==
  Bus Creator1 : BusCreator  Inputs=3
  vehBus_Values_BdyFrm_FrntAxl_Disp : Subsystem
  vehBus_Values_BdyFrm_FrntAxl_Steer : Subsystem
  vehBus_Values_BdyFrm_FrntAxl_Vel : Subsystem
  Out1 : Outport
  wires:
  vehBus_Values_BdyFrm_FrntAxl_Vel/1(Out1) -> Bus Creator1/2  "Vel"
  vehBus_Values_BdyFrm_FrntAxl_Steer/1(Out1) -> Bus Creator1/3  "Steer"
  vehBus_Values_BdyFrm_FrntAxl_Disp/1(Out1) -> Bus Creator1/1  "Disp"
  Bus Creator1/1 -> Out1/1

== system VehicleBody6DOFSSC/Body Sensor/BdyFrm/Moments ==
  Bus Creator2 : BusCreator  Inputs=3
  vehBus_Values_BdyFrm_Moments_Body : Subsystem
  vehBus_Values_BdyFrm_Moments_Drag : Subsystem
  vehBus_Values_BdyFrm_Moments_Ext : Subsystem
  Out1 : Outport
  wires:
  vehBus_Values_BdyFrm_Moments_Ext/1(Out1) -> Bus Creator2/3  "Ext"
  vehBus_Values_BdyFrm_Moments_Drag/1(Out1) -> Bus Creator2/2  "Drag"
  vehBus_Values_BdyFrm_Moments_Body/1(Out1) -> Bus Creator2/1  "Body"
  Bus Creator2/1 -> Out1/1

== system VehicleBody6DOFSSC/Body Sensor/BdyFrm/Pwr ==
  Drag : Constant  Value=zeros([1,1])  SampleTime=-1
  PwrExt : Constant  Value=zeros([1,1])  SampleTime=-1
  Signal Specification1 : SignalSpecification  Unit=W
  Signal Specification4 : SignalSpecification  Unit=W
  busOut : BusCreator  Inputs=2
  Out1 : Outport
  wires:
  busOut/1 -> Out1/1
  PwrExt/1 -> Signal Specification4/1  "PwrExt"
  Drag/1 -> Signal Specification1/1  "Drag"
  Signal Specification4/1 -> busOut/1  "PwrExt"
  Signal Specification1/1 -> busOut/2  "Drag"

== system VehicleBody6DOFSSC/Body Sensor/BdyFrm/RearAxl ==
  Bus Creator : BusCreator  Inputs=3
  vehBus_Values_BdyFrm_RearAxl_Disp : Subsystem
  vehBus_Values_BdyFrm_RearAxl_Steer : Subsystem
  vehBus_Values_BdyFrm_RearAxl_Vel : Subsystem
  Out1 : Outport
  wires:
  Bus Creator/1 -> Out1/1
  vehBus_Values_BdyFrm_RearAxl_Steer/1(Out1) -> Bus Creator/3  "Steer"
  vehBus_Values_BdyFrm_RearAxl_Vel/1(Out1) -> Bus Creator/2  "Vel"
  vehBus_Values_BdyFrm_RearAxl_Disp/1(Out1) -> Bus Creator/1  "Disp"

== system VehicleBody6DOFSSC/Body Sensor/InertFrm/Cg ==
  In : Inport
  Bus Creator4 : BusCreator  Inputs=3
  vehBus_Values_InertFrm_Cg_Ang : Subsystem
  vehBus_Values_InertFrm_Cg_Disp : Subsystem
  vehBus_Values_InertFrm_Cg_Vel : Subsystem
  Out1 : Outport
  wires:
  In/1 -> vehBus_Values_InertFrm_Cg_Vel/1(In), vehBus_Values_InertFrm_Cg_Disp/1(In), vehBus_Values_InertFrm_Cg_Ang/1(In)
  vehBus_Values_InertFrm_Cg_Disp/1(Out1) -> Bus Creator4/1  "Disp"
  vehBus_Values_InertFrm_Cg_Vel/1(Out1) -> Bus Creator4/2  "Vel"
  vehBus_Values_InertFrm_Cg_Ang/1(Out2) -> Bus Creator4/3  "Ang"
  Bus Creator4/1 -> Out1/1

== system VehicleBody6DOFSSC/Body Sensor/InertFrm/FrntAxl ==
  In : Inport
  Bus Creator : BusCreator  Inputs=2
  vehBus_Values_InertFrm_FrntAxl_Disp : Subsystem
  vehBus_Values_InertFrm_FrntAxl_Vel : Subsystem
  Out1 : Outport
  wires:
  vehBus_Values_InertFrm_FrntAxl_Disp/1(Out1) -> Bus Creator/1  "Disp"
  vehBus_Values_InertFrm_FrntAxl_Vel/1(Out1) -> Bus Creator/2  "Vel"
  Bus Creator/1 -> Out1/1
  In/1 -> vehBus_Values_InertFrm_FrntAxl_Disp/1(In), vehBus_Values_InertFrm_FrntAxl_Vel/1(In)

== system VehicleBody6DOFSSC/Body Sensor/InertFrm/Geom ==
  note: Assumes no Geometric
      | Simulation offsets
  In : Inport
  Bus Creator3 : BusCreator  Inputs=3
  vehBus_Values_InertFrm_Geom_Ang : Subsystem
  vehBus_Values_InertFrm_Geom_Disp : Subsystem
  vehBus_Values_InertFrm_Geom_Vel : Subsystem
  Out1 : Outport
  wires:
  Bus Creator3/1 -> Out1/1
  vehBus_Values_InertFrm_Geom_Vel/1(Out1) -> Bus Creator3/2  "Vel"
  vehBus_Values_InertFrm_Geom_Ang/1(Out1) -> Bus Creator3/3  "Ang"
  vehBus_Values_InertFrm_Geom_Disp/1(Out1) -> Bus Creator3/1  "Disp"
  In/1 -> vehBus_Values_InertFrm_Geom_Vel/1(In), vehBus_Values_InertFrm_Geom_Disp/1(In)

== system VehicleBody6DOFSSC/Body Sensor/InertFrm/Hitch ==
  Bus Creator2 : BusCreator  Inputs=2
  vehBus_Values_InertFrm_Hitch_Disp : Subsystem
  vehBus_Values_InertFrm_Hitch_Vel : Subsystem
  Out1 : Outport
  wires:
  vehBus_Values_InertFrm_Hitch_Disp/1(Out1) -> Bus Creator2/1  "Disp"
  vehBus_Values_InertFrm_Hitch_Vel/1(Out1) -> Bus Creator2/2  "Vel"
  Bus Creator2/1 -> Out1/1

== system VehicleBody6DOFSSC/Body Sensor/InertFrm/RearAxl ==
  RearAxl1 : Inport
  Bus Creator1 : BusCreator  Inputs=2
  vehBus_Values_InertFrm_RearAxl_Disp : Subsystem
  vehBus_Values_InertFrm_RearAxl_Vel : Subsystem
  Out1 : Outport
  wires:
  vehBus_Values_InertFrm_RearAxl_Disp/1(Out1) -> Bus Creator1/1  "Disp"
  vehBus_Values_InertFrm_RearAxl_Vel/1(Out1) -> Bus Creator1/2  "Vel"
  Bus Creator1/1 -> Out1/1
  RearAxl1/1 -> vehBus_Values_InertFrm_RearAxl_Disp/1(In), vehBus_Values_InertFrm_RearAxl_Vel/1(In)

== system VehicleBody6DOFSSC/Body Sensor/PwrInfo/vehBus_Values_PwrInfo_PwrNotTrnsfrd ==
  PwrFxDrag : Constant  Value=zeros([1,1])  SampleTime=-1
  Signal Specification5 : SignalSpecification  Unit=W
  busOut : BusCreator  Inputs=1
  Out1 : Outport
  wires:
  PwrFxDrag/1 -> busOut/1  "PwrFxDrag"
  busOut/1 -> Signal Specification5/1
  Signal Specification5/1 -> Out1/1

== system VehicleBody6DOFSSC/Body Sensor/PwrInfo/vehBus_Values_PwrInfo_PwrStored ==
  PwrStoredGrvty : Constant  Value=zeros([1,1])  SampleTime=-1
  PwrStoredxdot : Constant  Value=zeros([1,1])  SampleTime=-1
  Signal Specification5 : SignalSpecification  Unit=W
  busOut : BusCreator  Inputs=2
  Out1 : Outport
  wires:
  busOut/1 -> Signal Specification5/1
  PwrStoredGrvty/1 -> busOut/1  "PwrStoredGrvty"
  PwrStoredxdot/1 -> busOut/2  "PwrStoredxdot"
  Signal Specification5/1 -> Out1/1

== system VehicleBody6DOFSSC/Body Sensor/PwrInfo/vehBus_Values_PwrInfo_PwrTrnsfrd ==
  PwrFwFx : Constant  Value=zeros([1,1])  SampleTime=-1
  PwrFwRx : Constant  Value=zeros([1,1])  SampleTime=-1
  PwrFxExt : Constant  Value=zeros([1,1])  SampleTime=-1
  Signal Specification5 : SignalSpecification  Unit=W
  busOut : BusCreator  Inputs=3
  Out1 : Outport
  wires:
  PwrFwRx/1 -> busOut/3  "PwrFwRx"
  PwrFwFx/1 -> busOut/2  "PwrFwFx"
  PwrFxExt/1 -> busOut/1  "PwrFxExt"
  busOut/1 -> Signal Specification5/1
  Signal Specification5/1 -> Out1/1

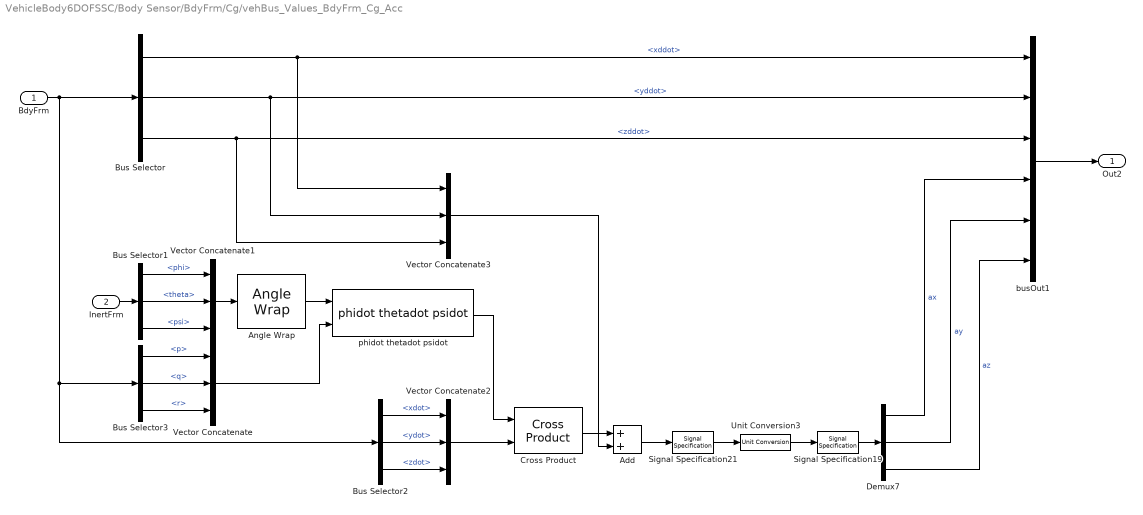
== system VehicleBody6DOFSSC/Body Sensor/BdyFrm/Cg/vehBus_Values_BdyFrm_Cg_Acc ==
  BdyFrm : Inport
  InertFrm : Inport  Port=2
  Add : Sum
  Angle Wrap : vehdynlibeomcommon/6 DOF Generic Vehicle Body/SignalCollection/Angle Wrap  SystemSampleTime=-1  VariantControl=Variant1  LabelModeActiveChoice=Unwrap  VariantActivationTime=update diagram  AllowFlexibleInterface=on  Latency=0  AutoFrameSizeCalculation=off
      link override Unwrap/Unwrap: aMode=6
  Bus Selector : BusSelector  OutputSignals=xddot,yddot,zddot
  Bus Selector1 : BusSelector  OutputSignals=phi,theta,psi
  Bus Selector2 : BusSelector  OutputSignals=xdot,ydot,zdot
  Bus Selector3 : BusSelector  OutputSignals=p,q,r
  Cross Product : matrix_library/Cross Product
  Demux7 : Demux  Outputs=3
  Signal Specification19 : SignalSpecification  Unit=gn
  Signal Specification21 : SignalSpecification  Unit=m/s^2
  Unit Conversion3 : UnitConversion
  Vector Concatenate{,1..3} (4 alike) : Concatenate  NumInputs=3
  busOut1 : BusCreator  Inputs=6
  phidot thetadot psidot : vehdynlibeomcommon/6 DOF Generic Vehicle Body/SignalCollection/phidot thetadot psidot  SystemSampleTime=-1  VariantActivationTime=update diagram  AllowFlexibleInterface=on  Latency=0  AutoFrameSizeCalculation=off
  Out2 : Outport
  wires:
  busOut1/1 -> Out2/1
  Bus Selector/3 -> Vector Concatenate3/3, busOut1/3  "<zddot>"
  Bus Selector/2 -> Vector Concatenate3/2, busOut1/2  "<yddot>"
  BdyFrm/1 -> Bus Selector/1, Bus Selector3/1, Bus Selector2/1
  Bus Selector/1 -> Vector Concatenate3/1, busOut1/1  "<xddot>"
  Vector Concatenate1/1 -> Angle Wrap/1
  Vector Concatenate/1 -> phidot thetadot psidot/2
  Angle Wrap/1 -> phidot thetadot psidot/1
  InertFrm/1 -> Bus Selector1/1
  Bus Selector3/1 -> Vector Concatenate/1  "<p>"
  Bus Selector3/2 -> Vector Concatenate/2  "<q>"
  Bus Selector3/3 -> Vector Concatenate/3  "<r>"
  Bus Selector1/3 -> Vector Concatenate1/3  "<psi>"
  Bus Selector1/2 -> Vector Concatenate1/2  "<theta>"
  Bus Selector1/1 -> Vector Concatenate1/1  "<phi>"
  phidot thetadot psidot/1 -> Cross Product/1
  Bus Selector2/1 -> Vector Concatenate2/1  "<xdot>"
  Bus Selector2/2 -> Vector Concatenate2/2  "<ydot>"
  Bus Selector2/3 -> Vector Concatenate2/3  "<zdot>"
  Vector Concatenate2/1 -> Cross Product/2
  Signal Specification21/1 -> Unit Conversion3/1
  Add/1 -> Signal Specification21/1
  Cross Product/1 -> Add/1
  Vector Concatenate3/1 -> Add/2
  Demux7/1 -> busOut1/4  "ax"
  Unit Conversion3/1 -> Signal Specification19/1
  Demux7/2 -> busOut1/5  "ay"
  Demux7/3 -> busOut1/6  "az"
  Signal Specification19/1 -> Demux7/1

== system VehicleBody6DOFSSC/Body Sensor/BdyFrm/Cg/vehBus_Values_BdyFrm_Cg_AngAcc ==
  In : Inport
  Bus Selector : BusSelector  OutputSignals=pdot,qdot,rdot
  busOut1 : BusCreator  Inputs=3
  Out2 : Outport
  wires:
  busOut1/1 -> Out2/1
  Bus Selector/3 -> busOut1/3  "<rdot>"
  Bus Selector/2 -> busOut1/2  "<qdot>"
  In/1 -> Bus Selector/1
  Bus Selector/1 -> busOut1/1  "<pdot>"

== system VehicleBody6DOFSSC/Body Sensor/BdyFrm/Cg/vehBus_Values_BdyFrm_Cg_AngVel ==
  In : Inport
  Bus Selector : BusSelector  OutputSignals=p,q,r
  busOut1 : BusCreator  Inputs=3
  Out2 : Outport
  wires:
  busOut1/1 -> Out2/1
  Bus Selector/3 -> busOut1/3  "<r>"
  Bus Selector/2 -> busOut1/2  "<q>"
  In/1 -> Bus Selector/1
  Bus Selector/1 -> busOut1/1  "<p>"

== system VehicleBody6DOFSSC/Body Sensor/BdyFrm/Cg/vehBus_Values_BdyFrm_Cg_Disp ==
  In : Inport
  Bus Selector : BusSelector  OutputSignals=x,y,z
  busOut1 : BusCreator  Inputs=3
  Out2 : Outport
  wires:
  busOut1/1 -> Out2/1
  Bus Selector/3 -> busOut1/3  "<z>"
  Bus Selector/2 -> busOut1/2  "<y>"
  In/1 -> Bus Selector/1
  Bus Selector/1 -> busOut1/1  "<x>"

== system VehicleBody6DOFSSC/Body Sensor/BdyFrm/Cg/vehBus_Values_BdyFrm_Cg_Vel ==
  In : Inport
  Bus Selector : BusSelector  OutputSignals=xdot,ydot,zdot
  busOut : BusCreator  Inputs=3
  Out1 : Outport
  wires:
  Bus Selector/3 -> busOut/3  "<zdot>"
  Bus Selector/2 -> busOut/2  "<ydot>"
  Bus Selector/1 -> busOut/1  "<xdot>"
  In/1 -> Bus Selector/1
  busOut/1 -> Out1/1

== system VehicleBody6DOFSSC/Body Sensor/BdyFrm/Forces/vehBus_Values_BdyFrm_Forces_Body ==
  Fx : Constant  Value=zeros([1,4526])  SampleTime=-1
  Fy : Constant  Value=zeros([1,1])  SampleTime=-1
  Fz : Constant  Value=zeros([1,1])  SampleTime=-1
  Signal Specification3 : SignalSpecification  Unit=N
  busOut : BusCreator  Inputs=3
  Out1 : Outport
  wires:
  Signal Specification3/1 -> Out1/1
  Fz/1 -> busOut/3  "Fz"
  Fx/1 -> busOut/1  "Fx"
  Fy/1 -> busOut/2  "Fy"
  busOut/1 -> Signal Specification3/1

== system VehicleBody6DOFSSC/Body Sensor/BdyFrm/Forces/vehBus_Values_BdyFrm_Forces_Drag ==
  Fx : Constant  Value=zeros([1,4526])  SampleTime=-1
  Fy : Constant  Value=zeros([1,1])  SampleTime=-1
  Fz : Constant  Value=zeros([1,1])  SampleTime=-1
  Signal Specification3 : SignalSpecification  Unit=N
  busOut : BusCreator  Inputs=3
  Out1 : Outport
  wires:
  Signal Specification3/1 -> Out1/1
  Fz/1 -> busOut/3  "Fz"
  Fx/1 -> busOut/1  "Fx"
  Fy/1 -> busOut/2  "Fy"
  busOut/1 -> Signal Specification3/1

== system VehicleBody6DOFSSC/Body Sensor/BdyFrm/Forces/vehBus_Values_BdyFrm_Forces_Ext ==
  Fx : Constant  Value=zeros([1,4526])  SampleTime=-1
  Fy : Constant  Value=zeros([1,1])  SampleTime=-1
  Fz : Constant  Value=zeros([1,1])  SampleTime=-1
  Signal Specification3 : SignalSpecification  Unit=N
  busOut : BusCreator  Inputs=3
  Out1 : Outport
  wires:
  Signal Specification3/1 -> Out1/1
  Fz/1 -> busOut/3  "Fz"
  Fx/1 -> busOut/1  "Fx"
  Fy/1 -> busOut/2  "Fy"
  busOut/1 -> Signal Specification3/1

== system VehicleBody6DOFSSC/Body Sensor/BdyFrm/Forces/vehBus_Values_BdyFrm_Forces_FrntAxl ==
  Fx : Constant  Value=zeros([1,4526])  SampleTime=-1
  Fy : Constant  Value=zeros([1,1])  SampleTime=-1
  Fz : Constant  Value=zeros([1,1])  SampleTime=-1
  Signal Specification3 : SignalSpecification  Unit=N
  busOut : BusCreator  Inputs=3
  Out1 : Outport
  wires:
  Fy/1 -> busOut/2  "Fy"
  busOut/1 -> Signal Specification3/1
  Fx/1 -> busOut/1  "Fx"
  Fz/1 -> busOut/3  "Fz"
  Signal Specification3/1 -> Out1/1

== system VehicleBody6DOFSSC/Body Sensor/BdyFrm/Forces/vehBus_Values_BdyFrm_Forces_Grvty ==
  Fx : Constant  Value=zeros([1,4526])  SampleTime=-1
  Fy : Constant  Value=zeros([1,1])  SampleTime=-1
  Fz : Constant  Value=zeros([1,1])  SampleTime=-1
  Signal Specification3 : SignalSpecification  Unit=N
  busOut : BusCreator  Inputs=3
  Out1 : Outport
  wires:
  Signal Specification3/1 -> Out1/1
  Fz/1 -> busOut/3  "Fz"
  Fx/1 -> busOut/1  "Fx"
  Fy/1 -> busOut/2  "Fy"
  busOut/1 -> Signal Specification3/1

== system VehicleBody6DOFSSC/Body Sensor/BdyFrm/Forces/vehBus_Values_BdyFrm_Forces_RearAxl ==
  Fx : Constant  Value=zeros([1,4526])  SampleTime=-1
  Fy : Constant  Value=zeros([1,1])  SampleTime=-1
  Fz : Constant  Value=zeros([1,1])  SampleTime=-1
  Signal Specification3 : SignalSpecification  Unit=N
  busOut : BusCreator  Inputs=3
  Out1 : Outport
  wires:
  Signal Specification3/1 -> Out1/1
  Fz/1 -> busOut/3  "Fz"
  Fx/1 -> busOut/1  "Fx"
  Fy/1 -> busOut/2  "Fy"
  busOut/1 -> Signal Specification3/1

== system VehicleBody6DOFSSC/Body Sensor/BdyFrm/Forces/vehBus_Values_BdyFrm_Forces_Tires_FrntTire ==
  Fx : Constant  Value=zeros([1,4526])  SampleTime=-1
  Fy : Constant  Value=zeros([1,1])  SampleTime=-1
  Fz : Constant  Value=zeros([1,1])  SampleTime=-1
  Signal Specification3 : SignalSpecification  Unit=N
  busOut : BusCreator  Inputs=3
  Out1 : Outport
  wires:
  Signal Specification3/1 -> Out1/1
  Fz/1 -> busOut/3  "Fz"
  Fx/1 -> busOut/1  "Fx"
  Fy/1 -> busOut/2  "Fy"
  busOut/1 -> Signal Specification3/1

== system VehicleBody6DOFSSC/Body Sensor/BdyFrm/Forces/vehBus_Values_BdyFrm_Forces_Tires_RearTire ==
  Fx : Constant  Value=zeros([1,4526])  SampleTime=-1
  Fy : Constant  Value=zeros([1,1])  SampleTime=-1
  Fz : Constant  Value=zeros([1,1])  SampleTime=-1
  Signal Specification3 : SignalSpecification  Unit=N
  busOut : BusCreator  Inputs=3
  Out1 : Outport
  wires:
  Signal Specification3/1 -> Out1/1
  Fz/1 -> busOut/3  "Fz"
  Fx/1 -> busOut/1  "Fx"
  Fy/1 -> busOut/2  "Fy"
  busOut/1 -> Signal Specification3/1

== system VehicleBody6DOFSSC/Body Sensor/BdyFrm/FrntAxl/vehBus_Values_BdyFrm_FrntAxl_Disp ==
  Signal Specification4 : SignalSpecification  Unit=m
  busOut : BusCreator  Inputs=3
  x : Constant  Value=zeros([1,1])  SampleTime=-1
  y : Constant  Value=zeros([1,1])  SampleTime=-1
  z : Constant  Value=zeros([1,1])  SampleTime=-1
  Out1 : Outport
  wires:
  z/1 -> busOut/3  "z"
  x/1 -> busOut/1  "x"
  y/1 -> busOut/2  "y"
  busOut/1 -> Signal Specification4/1
  Signal Specification4/1 -> Out1/1

== system VehicleBody6DOFSSC/Body Sensor/BdyFrm/FrntAxl/vehBus_Values_BdyFrm_FrntAxl_Steer ==
  Signal Specification4 : SignalSpecification  Unit=rad
  WhlAngFL : Constant  Value=zeros([1,1])  SampleTime=-1
  WhlAngFR : Constant  Value=zeros([1,1])  SampleTime=-1
  busOut : BusCreator  Inputs=2
  Out1 : Outport
  wires:
  busOut/1 -> Signal Specification4/1
  WhlAngFR/1 -> busOut/2  "WhlAngFR"
  WhlAngFL/1 -> busOut/1  "WhlAngFL"
  Signal Specification4/1 -> Out1/1

== system VehicleBody6DOFSSC/Body Sensor/BdyFrm/FrntAxl/vehBus_Values_BdyFrm_FrntAxl_Vel ==
  Signal Specification4 : SignalSpecification  Unit=m/s
  busOut : BusCreator  Inputs=3
  xdot : Constant  Value=zeros([1,1])  SampleTime=-1
  ydot : Constant  Value=zeros([1,1])  SampleTime=-1
  zdot : Constant  Value=zeros([1,1])  SampleTime=-1
  Out1 : Outport
  wires:
  zdot/1 -> busOut/3  "zdot"
  xdot/1 -> busOut/1  "xdot"
  ydot/1 -> busOut/2  "ydot"
  busOut/1 -> Signal Specification4/1
  Signal Specification4/1 -> Out1/1

== system VehicleBody6DOFSSC/Body Sensor/BdyFrm/Moments/vehBus_Values_BdyFrm_Moments_Body ==
  Mx : Constant  Value=zeros([1,1])  SampleTime=-1
  My : Constant  Value=zeros([1,1])  SampleTime=-1
  Mz : Constant  Value=zeros([1,1])  SampleTime=-1
  Signal Specification3 : SignalSpecification  Unit=N*m
  busOut : BusCreator  Inputs=3
  Out1 : Outport
  wires:
  My/1 -> busOut/2  "My"
  Mz/1 -> busOut/3  "Mz"
  Signal Specification3/1 -> Out1/1
  busOut/1 -> Signal Specification3/1
  Mx/1 -> busOut/1  "Mx"

== system VehicleBody6DOFSSC/Body Sensor/BdyFrm/Moments/vehBus_Values_BdyFrm_Moments_Drag ==
  Mx : Constant  Value=zeros([1,1])  SampleTime=-1
  My : Constant  Value=zeros([1,1])  SampleTime=-1
  Mz : Constant  Value=zeros([1,1])  SampleTime=-1
  Signal Specification3 : SignalSpecification  Unit=N*m
  busOut : BusCreator  Inputs=3
  Out1 : Outport
  wires:
  My/1 -> busOut/2  "My"
  Mz/1 -> busOut/3  "Mz"
  Signal Specification3/1 -> Out1/1
  busOut/1 -> Signal Specification3/1
  Mx/1 -> busOut/1  "Mx"

== system VehicleBody6DOFSSC/Body Sensor/BdyFrm/Moments/vehBus_Values_BdyFrm_Moments_Ext ==
  Mx : Constant  Value=zeros([1,1])  SampleTime=-1
  My : Constant  Value=zeros([1,1])  SampleTime=-1
  Mz : Constant  Value=zeros([1,1])  SampleTime=-1
  Signal Specification3 : SignalSpecification  Unit=N*m
  busOut : BusCreator  Inputs=3
  Out1 : Outport
  wires:
  Mz/1 -> busOut/3  "Mz"
  My/1 -> busOut/2  "My"
  busOut/1 -> Signal Specification3/1
  Mx/1 -> busOut/1  "Mx"
  Signal Specification3/1 -> Out1/1

== system VehicleBody6DOFSSC/Body Sensor/BdyFrm/RearAxl/vehBus_Values_BdyFrm_RearAxl_Disp ==
  Signal Specification4 : SignalSpecification  Unit=m
  busOut : BusCreator  Inputs=3
  x : Constant  Value=zeros([1,1])  SampleTime=-1
  y : Constant  Value=zeros([1,1])  SampleTime=-1
  z : Constant  Value=zeros([1,1])  SampleTime=-1
  Out1 : Outport
  wires:
  z/1 -> busOut/3  "z"
  busOut/1 -> Signal Specification4/1
  y/1 -> busOut/2  "y"
  x/1 -> busOut/1  "x"
  Signal Specification4/1 -> Out1/1

== system VehicleBody6DOFSSC/Body Sensor/BdyFrm/RearAxl/vehBus_Values_BdyFrm_RearAxl_Steer ==
  Signal Specification4 : SignalSpecification  Unit=rad
  WhlAngRL : Constant  Value=zeros([1,1])  SampleTime=-1
  WhlAngRR : Constant  Value=zeros([1,1])  SampleTime=-1
  busOut : BusCreator  Inputs=2
  Out1 : Outport
  wires:
  WhlAngRR/1 -> busOut/2  "WhlAngRR"
  WhlAngRL/1 -> busOut/1  "WhlAngRL"
  busOut/1 -> Signal Specification4/1
  Signal Specification4/1 -> Out1/1

== system VehicleBody6DOFSSC/Body Sensor/BdyFrm/RearAxl/vehBus_Values_BdyFrm_RearAxl_Vel ==
  Signal Specification4 : SignalSpecification  Unit=m/s
  busOut : BusCreator  Inputs=3
  xdot : Constant  Value=zeros([1,1])  SampleTime=-1
  ydot : Constant  Value=zeros([1,1])  SampleTime=-1
  zdot : Constant  Value=zeros([1,1])  SampleTime=-1
  Out1 : Outport
  wires:
  busOut/1 -> Signal Specification4/1
  ydot/1 -> busOut/2  "ydot"
  zdot/1 -> busOut/3  "zdot"
  xdot/1 -> busOut/1  "xdot"
  Signal Specification4/1 -> Out1/1

== system VehicleBody6DOFSSC/Body Sensor/InertFrm/Cg/vehBus_Values_InertFrm_Cg_Ang ==
  In : Inport
  Bus Selector : BusSelector  OutputSignals=phi,theta,psi
  busOut1 : BusCreator  Inputs=3
  Out2 : Outport
  wires:
  busOut1/1 -> Out2/1
  Bus Selector/3 -> busOut1/3  "<psi>"
  Bus Selector/2 -> busOut1/2  "<theta>"
  In/1 -> Bus Selector/1
  Bus Selector/1 -> busOut1/1  "<phi>"

== system VehicleBody6DOFSSC/Body Sensor/InertFrm/Cg/vehBus_Values_InertFrm_Cg_Disp ==
  In : Inport
  Bus Selector : BusSelector  OutputSignals=X,Y,Z
  busOut : BusCreator  Inputs=3
  Out1 : Outport
  wires:
  busOut/1 -> Out1/1
  In/1 -> Bus Selector/1
  Bus Selector/1 -> busOut/1  "<X>"
  Bus Selector/2 -> busOut/2  "<Y>"
  Bus Selector/3 -> busOut/3  "<Z>"

== system VehicleBody6DOFSSC/Body Sensor/InertFrm/Cg/vehBus_Values_InertFrm_Cg_Vel ==
  In : Inport
  Bus Selector : BusSelector  OutputSignals=Xdot,Ydot,Zdot
  busOut : BusCreator  Inputs=3
  Out1 : Outport
  wires:
  busOut/1 -> Out1/1
  In/1 -> Bus Selector/1
  Bus Selector/1 -> busOut/1  "<Xdot>"
  Bus Selector/2 -> busOut/2  "<Ydot>"
  Bus Selector/3 -> busOut/3  "<Zdot>"

== system VehicleBody6DOFSSC/Body Sensor/InertFrm/FrntAxl/vehBus_Values_InertFrm_FrntAxl_Disp ==
  In : Inport
  Bus Selector : BusSelector  OutputSignals=X,Y,Z
  busOut : BusCreator  Inputs=3
  Out1 : Outport
  wires:
  busOut/1 -> Out1/1
  Bus Selector/2 -> busOut/2  "<Y>"
  In/1 -> Bus Selector/1
  Bus Selector/3 -> busOut/3  "<Z>"
  Bus Selector/1 -> busOut/1  "<X>"

== system VehicleBody6DOFSSC/Body Sensor/InertFrm/FrntAxl/vehBus_Values_InertFrm_FrntAxl_Vel ==
  In : Inport
  Bus Selector : BusSelector  OutputSignals=Xdot,Ydot,Zdot
  busOut : BusCreator  Inputs=3
  Out1 : Outport
  wires:
  busOut/1 -> Out1/1
  Bus Selector/3 -> busOut/3  "<Zdot>"
  Bus Selector/2 -> busOut/2  "<Ydot>"
  Bus Selector/1 -> busOut/1  "<Xdot>"
  In/1 -> Bus Selector/1
